simulink model "full_system"  (R2023b)
settings: Solver=VariableStepAuto  StartTime=0.0  StopTime=0.5  RelTol=1e-3
InitFcn:
  | init_full;
StopFcn:
  | PlotResults;
values from neighbouring files (symbols this model uses):
  Co = DCDC_Co*(10^-6)    [init_full.m]
  enc_offset = rand*2*pi    [init_full.m]
  id_KtMax = [0 -0.537821267309 -1.89621818766 -3.99825634278 -6.70443962951 -9.96764643107 -13.6215947621 -17.6528328359 -21.9311457912 -26.4320408854 -31.0887852115 -35.9145699207 ... (100 elements, 1x100)]    [Data_DCDC_converter.mat]
  IinMax = I_in_rated    [init_full.m]
  Imax = I_max    [init_full.m]
  iq_KtMax = [0 7.75916074359 15.4395487378 22.9882228687 30.3801205367 37.5897819046 44.6344030308 51.5031554736 58.229114561 64.8178001373 71.2942504703 77.6524098392 ... (100 elements, 1x100)]    [Data_DCDC_converter.mat]
  kid = 0.05*kpd*wb    [init_full.m]
  kii = 2106.71507358    [Data_DCDC_converter.mat]    (also in init_full.m = wzi*kpi)
  kiq = 0.05*kpq*wb    [init_full.m]
  kiv = 443.093490604    [Data_DCDC_converter.mat]    (also in init_full.m = kpv*wzv)
  kpd = wb*ld    [init_full.m]
  kpi = 1.75559589465    [Data_DCDC_converter.mat]    (also in init_full.m = wci*Lin)
  kpq = wb*lq    [init_full.m]
  kpv = 0.678584013175    [Data_DCDC_converter.mat]    (also in init_full.m = wcv*Co)
  lambda_m = F_m    [init_full.m]
  Lin = L    [init_full.m]
  p = 3    [Data_DCDC_converter.mat]
  Rs = 0.05    [Data_DCDC_converter.mat]
  Tau_d = 1.5*Ts    [init_full.m]
  TimeEnable = 5e-3    (= 0.005)    [init_full.m]
  Trise = 25e-3    (= 0.025)    [init_full.m]
  Ts = 1/fs    [init_full.m]
  Ts_inv = 1/fs_inv    [init_full.m]
  Vbat = DCDC_vbatt    [init_full.m]
  Vdc = Vdc_max    [init_full.m]
  VdcSetpoint = Vdc_max    [init_full.m]
  w_mech = 2459    [init_full.m]
undefined symbols (not defined in the file or in its folder): DiscIntNeverNeededParam, Ld_nom, Lq_nom, sigbuilder_block, T_KtMax
libraries: simulink x6, spsMeanLib x1
settings Model: Creator=giuse  LastModifiedBy=giuse

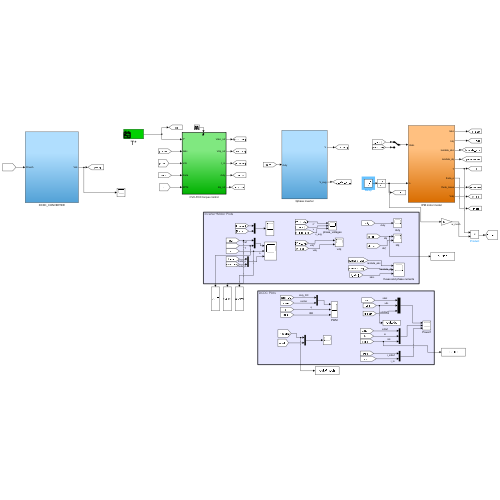
[thumbnail: Simulink's stored preview of the top-level diagram]
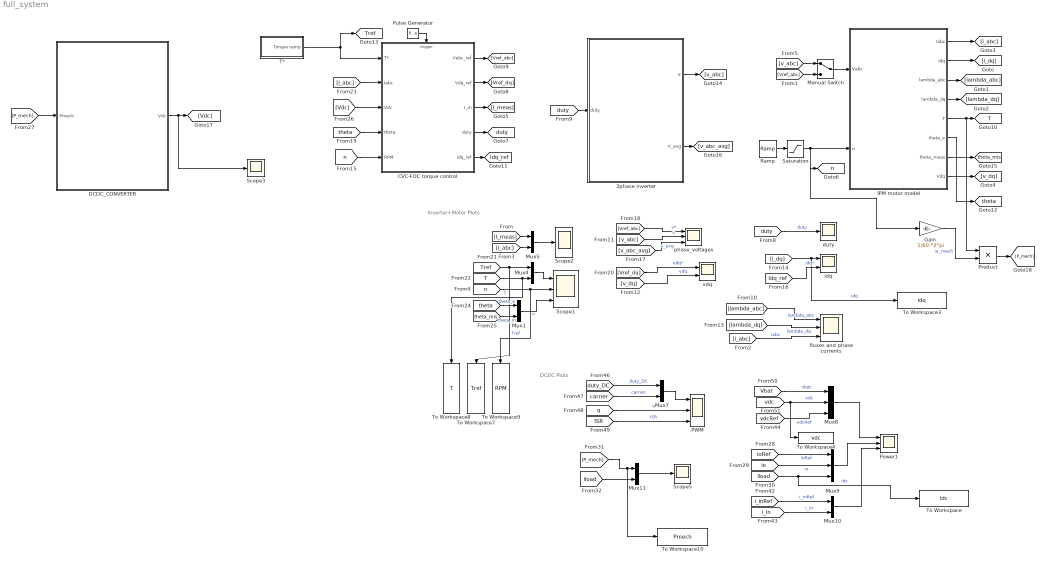
== system full_system ==
  note: DCDC Plots
  note: Inverter+Motor Plots
  3phase inverter : Subsystem
  CVC-FOC torque control : Subsystem
  DCDC_CONVERTER : Subsystem
  Gain : Gain  Gain=1/60 *2*pi
  IPM motor model : Subsystem
  Manual Switch : ManualSwitch
  Mux{1,4..5,7,10..11} (6 alike) : Mux  Inputs=2
  Mux8 : Mux  Inputs=3
  Mux9 : Mux  Inputs=3
  PWM : Scope  NumInputPorts=3
  Power1 : Scope  NumInputPorts=3
  Product : Product
  Pulse Generator : DiscretePulseGenerator  PulseType=Time based  Period=Ts_inv  PulseWidth=20
  Ramp : simulink/Sources/Ramp  slope=w_mech/0.3  start=0.1  InitialOutput=0
  Saturation : Saturate  UpperLimit=w_mech  LowerLimit=-100
  Scope1 : Scope  NumInputPorts=3
  Scope2 : Scope
  Scope3 : Scope
  Scope5 : Scope
  T* : Subsystem  Tag=STV Subsys  LoadFcn=sigbuilder_block('load');  StartFcn=sigbuilder_block('start');  StopFcn=sigbuilder_block('stop');  ClipboardFcn=sigbuilder_block('clipboard');  mask(Sigbuilder block){tuvar=[0:10]}
      mask help: Simulink:masks:SigbuilderBlock_MD
      mask init:
      | if ~strcmp(get_param(bdroot(gcbh),'SimulationStatus'),'stopped') tuvar = sigbuilder_block('maskInit'); end
      settings: CopyFcn=sigbuilder_block('copy');  DeleteFcn=sigbuilder_block('delete');  ModelCloseFcn=sigbuilder_block('modelClose');  PreSaveFcn=sigbuilder_block('preSave');  PauseFcn=sigbuilder_block('pause');  ContinueFcn=sigbuilder_block('continue');  NameChangeFcn=sigbuilder_block('namechange');  OpenFcn=sigbuilder_block('open',[5.4 30 1141.2 522.6 ]);  CloseFcn=sigbuilder_block('close');
      mask Display: plot(0, 0, 100, 100,[2, 2, 32, 32, 2], [68, 8, 8, 68, 68],[32, 2], [38, 38], [32, 19, 2],[53, 60, 44], [32, 17, 17, 2],[16, 16, 31, 31]);txt = getActiveGroup(gcbh);text(2, 100, txt,'verticalAlignment', 'top');
  To Workspace : ToWorkspace  VariableName=idc  SampleTime=-1
  To Workspace10 : ToWorkspace  VariableName=Pmech  SampleTime=-1
  To Workspace3 : ToWorkspace  VariableName=idq  SampleTime=-1
  To Workspace4 : ToWorkspace  VariableName=vdc  SampleTime=-1
  To Workspace7 : ToWorkspace  VariableName=Tref  SampleTime=-1
  To Workspace8 : ToWorkspace  VariableName=T  SampleTime=-1
  To Workspace9 : ToWorkspace  VariableName=RPM  SampleTime=-1
  duty : Scope
  fluxes and phase currents : Scope  NumInputPorts=3
  idq : Scope  NumInputPorts=2
  phase_voltages : Scope  NumInputPorts=3
  vdq : Scope  NumInputPorts=2
  tag scope: Idq_ref=global, T=global, Tref=global, duty=global, n=global, theta=global, theta_mis=global
  wires:
  [i_abc] -> CVC-FOC torque control/2(Iabc)
  [Vref_abc] -> phase_voltages/1  "v*"
  Pulse Generator/1 -> CVC-FOC torque control/Trigger
  CVC-FOC torque control/3(I_m) -> [I_meas]
  [v_abc] -> Manual Switch/1
  CVC-FOC torque control/5(Idq_ref) -> [Idq_ref]
  T*/1(Torque ramp) -> CVC-FOC torque control/1(T*), [Tref]
  IPM motor model/3(lambda_abc) -> [lambda_abc]
  CVC-FOC torque control/4(duty) -> [duty]
  [n] -> CVC-FOC torque control/5(RPM)
  [Idq_ref] -> idq/2  "idq*"
  [T] -> To Workspace8/1, Mux4/2  "T"
  [Vref_dq] -> vdq/1  "vdq*"
  [I_meas] -> Mux5/1
  3phase inverter/2(V_avg) -> [v_abc_avg]
  [i_dq] -> To Workspace3/1, idq/1  "idq"
  Manual Switch/1 -> IPM motor model/1(Vabc)
  [Vdc] -> CVC-FOC torque control/3(Vdc)
  Mux5/1 -> Scope2/1
  IPM motor model/1(Iabc) -> [i_abc]
  [i_abc] -> Mux5/2
  [Vref_abc] -> Manual Switch/2
  IPM motor model/8(Vdq) -> [v_dq]
  Mux4/1 -> Scope1/1
  CVC-FOC torque control/2(Vdq_ref) -> [Vref_dq]
  Saturation/1 -> [n], IPM motor model/2(n), Gain/1
  [v_abc] -> phase_voltages/2  "v"
  [Tref] -> Mux4/1, To Workspace7/1  "Tref"
  Ramp/1 -> Saturation/1
  [theta] -> CVC-FOC torque control/4(theta)
  IPM motor model/7(theta_meas) -> [theta_mis]
  IPM motor model/2(Idq) -> [i_dq]
  [theta_mis] -> Mux1/2  "theta_m"
  [duty] -> 3phase inverter/1(duty)
  CVC-FOC torque control/1(Vabc_ref) -> [Vref_abc]
  IPM motor model/6(theta_e) -> [theta]
  IPM motor model/5(T) -> Product/1, [T]
  [v_abc_avg] -> phase_voltages/3  "v_avg"
  [lambda_dq] -> fluxes and phase currents/2  "lambda_dq"
  [n] -> Scope1/2, To Workspace9/1  "n"
  [theta] -> Mux1/1  "theta_e"
  Mux1/1 -> Scope1/3
  IPM motor model/4(lambda_dq) -> [lambda_dq]
  3phase inverter/1(V) -> [v_abc]
  [v_dq] -> vdq/2  "vdq"
  [duty] -> duty/1  "duty"
  [lambda_abc] -> fluxes and phase currents/1  "lambda_abc"
  [i_abc] -> fluxes and phase currents/3  "iabc"
  Mux10/1 -> Power1/3
  [ioRef] -> Mux9/1  "ioRef"
  Mux7/1 -> PWM/1
  [i_inRef] -> Mux10/1  "i_inRef"
  [i_in] -> Mux10/2  "i_in"
  [carrier] -> Mux7/2  "carrier"
  [vdcRef] -> Mux8/3  "vdcRef"
  [ISR] -> PWM/3  "ISR"
  [Vbat] -> Mux8/1  "vbat"
  [q] -> PWM/2  "q"
  [iload] -> Mux9/3, To Workspace/1  "idc"
  [io] -> Mux9/2  "io"
  [vdc] -> To Workspace4/1, Mux8/2  "vdc"
  Mux8/1 -> Power1/1
  [duty_DC] -> Mux7/1  "duty_DC"
  Mux9/1 -> Power1/2
  DCDC_CONVERTER/1(Vdc) -> Scope3/1, [Vdc]
  Gain/1 -> Product/2  "w_mech"
  Product/1 -> [P_mech]
  [P_mech] -> DCDC_CONVERTER/1(Pmech)
  Mux11/1 -> Scope5/1
  [iload] -> Mux11/2
  [P_mech] -> To Workspace10/1, Mux11/1

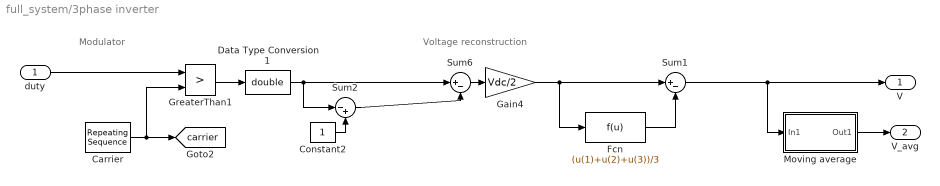
== system full_system/3phase inverter ==
  note: Modulator
  note: Voltage reconstruction
  duty : Inport
  Carrier : simulink/Sources/Repeating Sequence  rep_seq_t=[0 Ts/2 Ts]  rep_seq_y=[0 1 0]
  Constant2 : Constant
  Data Type Conversion1 : DataTypeConversion  OutDataTypeStr=double  SaturateOnIntegerOverflow=off  RndMeth=Floor
  Fcn : Fcn  Expr=(u(1)+u(2)+u(3))/3
  Gain4 : Gain  Gain=Vdc/2
  GreaterThan1 : RelationalOperator  Operator=>  OutDataTypeStr=boolean  RndMeth=Simplest  InputSameDT=off
  Moving average : Subsystem
  Sum1 : Sum  Inputs=|+-
  Sum2 : Sum  Inputs=|-+
  Sum6 : Sum  Inputs=|+-
  V : Outport  VectorParamsAs1DForOutWhenUnconnected=off
  V_avg : Outport  Port=2  VectorParamsAs1DForOutWhenUnconnected=off
  tag scope: carrier=global
  wires:
  GreaterThan1/1 -> Data Type Conversion1/1
  Moving average/1(Out1) -> V_avg/1
  Carrier/1 -> [carrier], GreaterThan1/2
  Data Type Conversion1/1 -> Sum2/1, Sum6/1
  Constant2/1 -> Sum2/2
  Sum6/1 -> Gain4/1
  duty/1 -> GreaterThan1/1
  Gain4/1 -> Fcn/1, Sum1/1
  Sum1/1 -> Moving average/1(In1), V/1
  Fcn/1 -> Sum1/2
  Sum2/1 -> Sum6/2

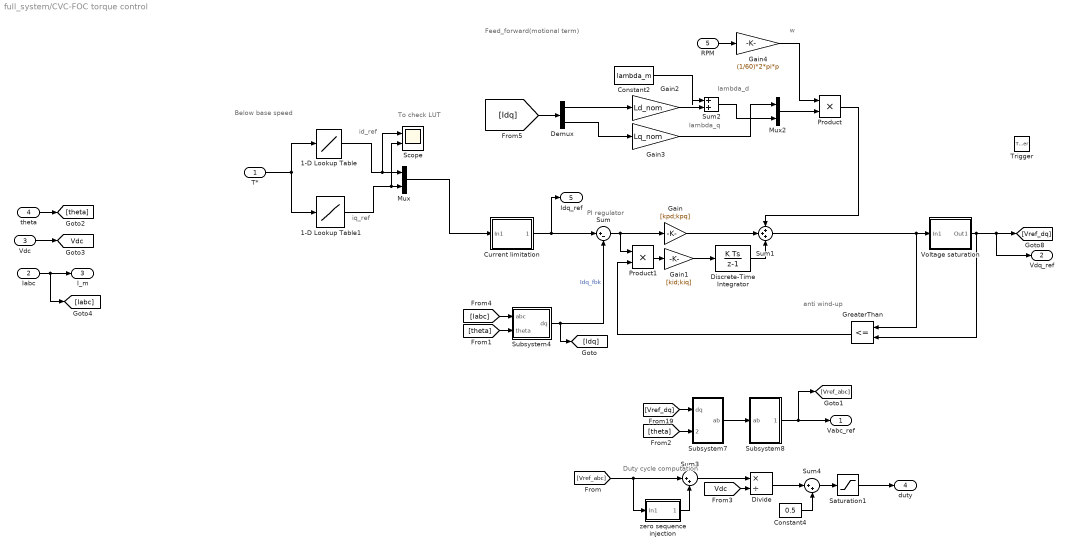
== system full_system/CVC-FOC torque control ==
  note: To check LUT
  note: Feed_forward(motional term)
  note: w
  note: lambda_q
  note: lambda_d
  note: iq_ref
  note: id_ref
  note: Below base speed
  note: anti wind-up
  note: PI regulator
  note: Duty cycle computation
  T* : Inport
  Iabc : Inport  Port=2
  Vdc : Inport  Port=3
  theta : Inport  Port=4
  RPM : Inport  Port=5
  Trigger : TriggerPort  VariantControl=Variant  PortDimensions=1
  1-D Lookup Table : Lookup_n-D  NumberOfTableDimensions=1  BreakpointsForDimension1=T_KtMax  Table=id_KtMax  InternalRulePriority=Speed  RndMeth=Simplest
  1-D Lookup Table1 : Lookup_n-D  NumberOfTableDimensions=1  BreakpointsForDimension1=T_KtMax  Table=iq_KtMax  InternalRulePriority=Speed  RndMeth=Simplest
  Constant2 : Constant  Value=lambda_m
  Constant4 : Constant  Value=0.5
  Current limitation : Subsystem
  Demux : Demux  Outputs=2
  Discrete-Time Integrator : DiscreteIntegrator  gainval=1  SampleTime=-1  ICPrevOutput=DiscIntNeverNeededParam  ICPrevScaledInput=DiscIntNeverNeededParam
  Divide : Product  Inputs=*/
  Gain : Gain  Gain=[kpd;kpq]
  Gain1 : Gain  Gain=[kid;kiq]
  Gain2 : Gain  Gain=Ld_nom
  Gain3 : Gain  Gain=Lq_nom
  Gain4 : Gain  Gain=(1/60)*2*pi*p
  GreaterThan : RelationalOperator  Operator=<=  OutDataTypeStr=boolean  RndMeth=Simplest  InputSameDT=off
  Mux : Mux  Inputs=2
  Mux2 : Mux  Inputs=2
  Product : Product
  Product1 : Product
  Saturation1 : Saturate  UpperLimit=1  LowerLimit=0
  Scope : Scope  NumInputPorts=2
  Subsystem4 : Subsystem
  Subsystem7 : Subsystem
  Subsystem8 : Subsystem
  Sum : Sum  Inputs=|+-
  Sum1 : Sum  Inputs=+++
  Sum2 : Sum  Inputs=|++
  Sum3 : Sum  Inputs=|++
  Sum4 : Sum  Inputs=|++
  Voltage saturation : Subsystem
  zero sequence injection : Subsystem
  Vabc_ref : Outport  VectorParamsAs1DForOutWhenUnconnected=off
  Vdq_ref : Outport  Port=2  VectorParamsAs1DForOutWhenUnconnected=off
  I_m : Outport  Port=3  VectorParamsAs1DForOutWhenUnconnected=off
  duty : Outport  Port=4  VectorParamsAs1DForOutWhenUnconnected=off
  Idq_ref : Outport  Port=5
  tag scope: Vdc=global
  wires:
  Subsystem7/1(ab) -> Subsystem8/1(ab)
  [Vref_dq] -> Subsystem7/1(dq)
  Subsystem8/1(abc) -> [Vref_abc], Vabc_ref/1
  Iabc/1 -> [Iabc], I_m/1
  Sum/1 -> Product1/1, Gain/1
  Gain1/1 -> Discrete-Time Integrator/1
  Saturation1/1 -> duty/1
  Constant4/1 -> Sum4/2
  zero sequence injection/1(Out1) -> Sum3/2
  Sum3/1 -> Divide/1
  [Vdc] -> Divide/2
  Sum4/1 -> Saturation1/1
  [Vref_abc] -> zero sequence injection/1(In1), Sum3/1
  Divide/1 -> Sum4/1
  theta/1 -> [theta]
  [theta] -> Subsystem7/2(theta)
  Subsystem4/1(dq) -> Sum/2, [Idq]  "Idq_fbk"
  Vdc/1 -> [Vdc]
  [theta] -> Subsystem4/2(theta)
  [Iabc] -> Subsystem4/1(abc)
  Sum1/1 -> Voltage saturation/1(In1), GreaterThan/1
  Product1/1 -> Gain1/1
  GreaterThan/1 -> Product1/2
  T*/1 -> 1-D Lookup Table1/1, 1-D Lookup Table/1
  1-D Lookup Table/1 -> Scope/1, Mux/1
  1-D Lookup Table1/1 -> Scope/2, Mux/2
  Current limitation/1(Idq_ref) -> Idq_ref/1, Sum/1
  Mux/1 -> Current limitation/1(In1)
  [Idq] -> Demux/1
  Demux/1 -> Gain2/1
  Gain2/1 -> Sum2/2
  Constant2/1 -> Sum2/1
  Demux/2 -> Gain3/1
  Sum2/1 -> Mux2/2
  Gain3/1 -> Mux2/1
  Mux2/1 -> Product/2
  RPM/1 -> Gain4/1
  Gain4/1 -> Product/1
  Discrete-Time Integrator/1 -> Sum1/3
  Gain/1 -> Sum1/2
  Product/1 -> Sum1/1
  Voltage saturation/1(Out1) -> [Vref_dq], Vdq_ref/1, GreaterThan/2

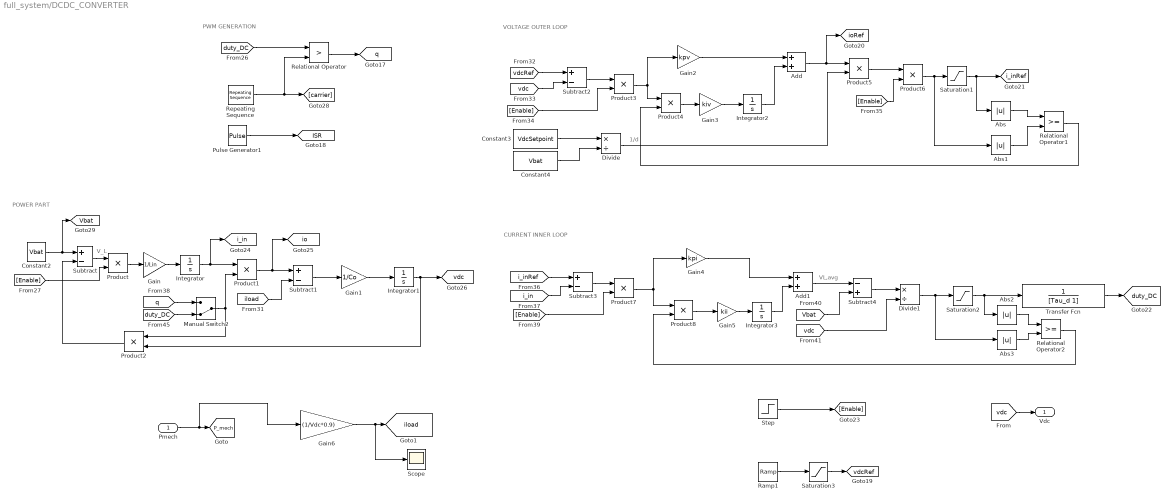
== system full_system/DCDC_CONVERTER ==
  note: V_L
  note: POWER PART
  note: PWM GENERATION
  note: CURRENT INNER LOOP
  note: VOLTAGE OUTER LOOP
  note: 1/d
  note: VL,avg
  Pmech : Inport
  Abs{,1..3} (4 alike) : Abs  SaturateOnIntegerOverflow=off
  Add : Sum
  Add1 : Sum
  Constant2 : Constant  Value=Vbat
  Constant3 : Constant  Value=VdcSetpoint
  Constant4 : Constant  Value=Vbat
  Divide : Product  Inputs=*/
  Divide1 : Product  Inputs=*/
  Gain : Gain  Gain=1/Lin
  Gain1 : Gain  Gain=1/Co
  Gain2 : Gain  Gain=kpv
  Gain3 : Gain  Gain=kiv
  Gain4 : Gain  Gain=kpi
  Gain5 : Gain  Gain=kii
  Gain6 : Gain  Gain=(1/Vdc*0.9)
  Integrator : Integrator
  Integrator1 : Integrator  InitialCondition=Vbat
  Integrator2 : Integrator
  Integrator3 : Integrator
  Manual Switch2 : ManualSwitch  CurrentSetting=0
  Product{,1..8} (9 alike) : Product
  Pulse Generator1 : DiscretePulseGenerator  PulseType=Time based  Period=Ts  PulseWidth=50
  Ramp1 : simulink/Sources/Ramp  slope=(VdcSetpoint-Vbat)/Trise  start=TimeEnable  InitialOutput=Vbat
  Relational Operator : RelationalOperator  Operator=>  RndMeth=Simplest  InputSameDT=off
  Relational Operator1 : RelationalOperator  RndMeth=Simplest
  Relational Operator2 : RelationalOperator  RndMeth=Simplest
  Repeating Sequence : simulink/Sources/Repeating Sequence  rep_seq_t=[0 Ts/2 Ts]  rep_seq_y=[0 1 0]
  Saturation1 : Saturate  UpperLimit=IinMax  LowerLimit=-IinMax
  Saturation2 : Saturate  UpperLimit=1  LowerLimit=0.1
  Saturation3 : Saturate  UpperLimit=VdcSetpoint  LowerLimit=Vbat
  Scope : Scope
  Step : Step  Time=TimeEnable  SampleTime=0
  Subtract{,1..3} (4 alike) : Sum  Inputs=+-
  Subtract4 : Sum  Inputs=-+
  Transfer Fcn : TransferFcn  Denominator=[Tau_d 1]
  Vdc : Outport
  tag scope: ISR=global, P_mech=global, Vbat=global, duty_DC=global, i_in=global, i_inRef=global, iload=global, io=global, ioRef=global, q=global, vdc=global, vdcRef=global
  wires:
  Transfer Fcn/1 -> [duty_DC]
  Manual Switch2/1 -> Product2/1, Product1/2
  Integrator1/1 -> [vdc], Product2/2
  Add1/1 -> Subtract4/1
  Subtract/1 -> Product/1
  Saturation3/1 -> [vdcRef]
  Saturation2/1 -> Transfer Fcn/1, Abs2/1
  Product6/1 -> Abs1/1, Saturation1/1
  Abs1/1 -> Relational Operator1/2
  [Enable] -> Product/2
  Subtract2/1 -> Product3/1
  Gain1/1 -> Integrator1/1
  Relational Operator2/1 -> Product8/2
  [Vbat] -> Subtract4/2
  Constant2/1 -> [Vbat], Subtract/1
  [i_inRef] -> Subtract3/1
  Subtract3/1 -> Product7/1
  Subtract1/1 -> Gain1/1
  Divide/1 -> Product5/2
  Product4/1 -> Gain3/1
  [i_in] -> Subtract3/2
  Ramp1/1 -> Saturation3/1
  Gain3/1 -> Integrator2/1
  Gain2/1 -> Add/1
  Constant3/1 -> Divide/1
  Integrator/1 -> Product1/1, [i_in]
  Subtract4/1 -> Divide1/1
  Pulse Generator1/1 -> [ISR]
  Product1/1 -> [io], Subtract1/1
  Product2/1 -> Subtract/2
  Gain/1 -> Integrator/1
  Product8/1 -> Gain5/1
  Product7/1 -> Product8/1, Gain4/1
  [duty_DC] -> Manual Switch2/2
  Divide1/1 -> Abs3/1, Saturation2/1
  [q] -> Manual Switch2/1
  [Enable] -> Product7/2
  [iload] -> Subtract1/2
  Relational Operator1/1 -> Product4/2
  [vdcRef] -> Subtract2/1
  Gain4/1 -> Add1/1
  [vdc] -> Divide1/2
  Repeating Sequence/1 -> [carrier], Relational Operator/2
  Abs3/1 -> Relational Operator2/2
  Product/1 -> Gain/1
  Relational Operator/1 -> [q]
  Abs/1 -> Relational Operator1/1
  [duty_DC] -> Relational Operator/1
  Abs2/1 -> Relational Operator2/1
  [Enable] -> Product6/2
  Gain5/1 -> Integrator3/1
  Step/1 -> [Enable]
  Integrator3/1 -> Add1/2
  Add/1 -> [ioRef], Product5/1
  Product5/1 -> Product6/1
  [vdc] -> Subtract2/2
  Saturation1/1 -> Abs/1, [i_inRef]
  Integrator2/1 -> Add/2
  Product3/1 -> Product4/1, Gain2/1
  [Enable] -> Product3/2
  Constant4/1 -> Divide/2
  [vdc] -> Vdc/1
  Pmech/1 -> Gain6/1, [P_mech]
  Gain6/1 -> Scope/1, [iload]

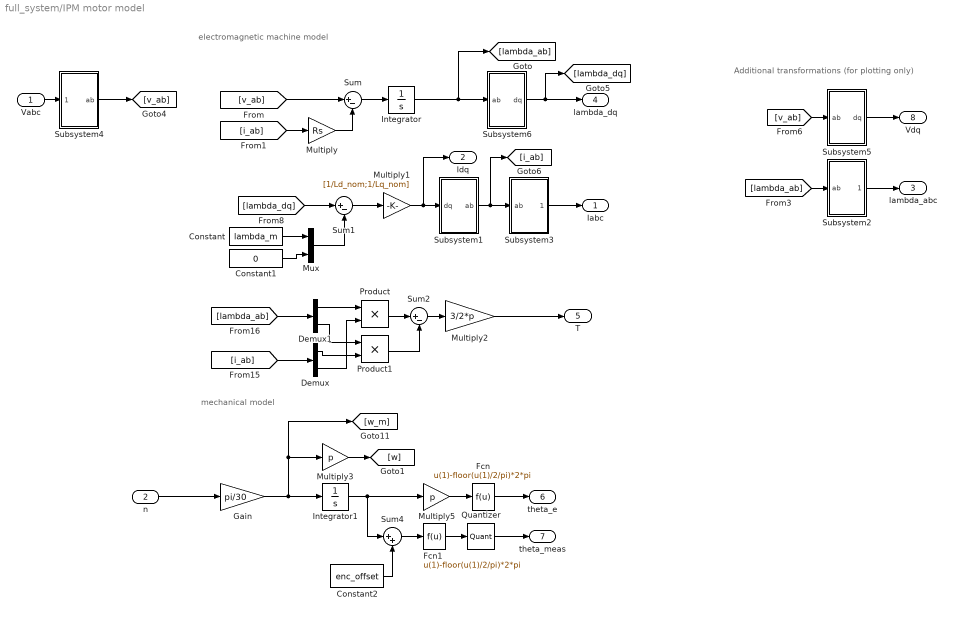
== system full_system/IPM motor model ==
  note: Additional transformations (for plotting only)
  note: mechanical model
  note: electromagnetic machine model
  Vabc : Inport
  n : Inport  Port=2
  Constant : Constant  Value=lambda_m
  Constant1 : Constant  Value=0
  Constant2 : Constant  Value=enc_offset
  Demux : Demux  Outputs=2
  Demux1 : Demux  Outputs=2
  Fcn : Fcn  Expr=u(1)-floor(u(1)/2/pi)*2*pi
  Fcn1 : Fcn  Expr=u(1)-floor(u(1)/2/pi)*2*pi
  Gain : Gain  Gain=pi/30
  Integrator : Integrator  InitialCondition=[lambda_m 0]
  Integrator1 : Integrator
  Multiply : Gain  Gain=Rs
  Multiply1 : Gain  Gain=[1/Ld_nom;1/Lq_nom]
  Multiply2 : Gain  Gain=3/2*p
  Multiply3 : Gain  Gain=p
  Multiply5 : Gain  Gain=p
  Mux : Mux  Inputs=2
  Product : Product
  Product1 : Product
  Quantizer : Quantizer  QuantizationInterval=2*pi/2048
  Subsystem1 : Subsystem
  Subsystem2 : Subsystem
  Subsystem3 : Subsystem
  Subsystem4 : Subsystem
  Subsystem5 : Subsystem
  Subsystem6 : Subsystem
  Sum : Sum  Inputs=|+-
  Sum1 : Sum  Inputs=|+-
  Sum2 : Sum  Inputs=|+-
  Sum4 : Sum  Inputs=|++
  Iabc : Outport  VectorParamsAs1DForOutWhenUnconnected=off
  Idq : Outport  Port=2  VectorParamsAs1DForOutWhenUnconnected=off
  lambda_abc : Outport  Port=3  VectorParamsAs1DForOutWhenUnconnected=off
  lambda_dq : Outport  Port=4  VectorParamsAs1DForOutWhenUnconnected=off
  T : Outport  Port=5  VectorParamsAs1DForOutWhenUnconnected=off
  theta_e : Outport  Port=6  VectorParamsAs1DForOutWhenUnconnected=off
  theta_meas : Outport  Port=7  VectorParamsAs1DForOutWhenUnconnected=off
  Vdq : Outport  Port=8  VectorParamsAs1DForOutWhenUnconnected=off
  wires:
  Integrator1/1 -> Multiply5/1, Sum4/1
  [v_ab] -> Sum/1
  [i_ab] -> Demux/1
  Fcn1/1 -> Quantizer/1
  [lambda_ab] -> Demux1/1
  Multiply/1 -> Sum/2
  Quantizer/1 -> theta_meas/1
  Integrator/1 -> Subsystem6/1(ab), [lambda_ab]
  Sum/1 -> Integrator/1
  Product/1 -> Sum2/1
  Subsystem4/1(ab) -> [v_ab]
  Subsystem6/1(dq) -> [lambda_dq], lambda_dq/1
  [lambda_dq] -> Sum1/1
  Subsystem5/1(dq) -> Vdq/1
  Sum1/1 -> Multiply1/1
  [v_ab] -> Subsystem5/1(ab)
  Fcn/1 -> theta_e/1
  Product1/1 -> Sum2/2
  Vabc/1 -> Subsystem4/1(abc)
  Multiply5/1 -> Fcn/1
  Subsystem1/1(ab) -> Subsystem3/1(ab), [i_ab]
  Multiply1/1 -> Idq/1, Subsystem1/1(dq)
  Sum4/1 -> Fcn1/1
  Gain/1 -> Integrator1/1, Multiply3/1, [w_m]
  Demux1/1 -> Product/1
  Demux/2 -> Product/2
  Demux1/2 -> Product1/1
  [lambda_ab] -> Subsystem2/1(ab)
  Demux/1 -> Product1/2
  [i_ab] -> Multiply/1
  Constant/1 -> Mux/1
  Constant1/1 -> Mux/2
  Mux/1 -> Sum1/2
  Sum2/1 -> Multiply2/1
  Constant2/1 -> Sum4/2
  Multiply2/1 -> T/1
  Subsystem3/1(abc) -> Iabc/1
  Subsystem2/1(abc) -> lambda_abc/1
  n/1 -> Gain/1
  Multiply3/1 -> [w]

== system full_system/T* ==
  Demux : Demux  Tag=STV Demux  Outputs=1
      settings: DisplayOption=none
  FromWs : FromWorkspace  Tag=STV FromWs  VariableName=tuvar
      SigBuilderData=|
      | common.afterFinalStr = 'Extrapolate'
      | common.sampleTime = 0
      | dataSet.timeRange = [0 3]
      | dataSet.name = 'T*'
      | sbobj.Groups.Name = 'T*'
      | sbobj.Groups.Signals.Name = 'Torque ramp'
      | sbobj.Groups.Signals.XData = [0 0.3 0.3 3]
      | sbobj.Groups.Signals.YData = [0 100 100 100]
      | sbobj.Groups.TimeRange = [0 3]
  Torque ramp : Outport  Tag=STV Outport
  wires:
  FromWs/1 -> Demux/1
  Demux/1 -> Torque ramp/1

== system full_system/3phase inverter/Moving average ==
  In1 : Inport
  Mean1 : spsMeanLib/Mean  Freq=fs  Vinit=0  Ts=0
  Out1 : Outport  VectorParamsAs1DForOutWhenUnconnected=off
  wires:
  In1/1 -> Mean1/1
  Mean1/1 -> Out1/1

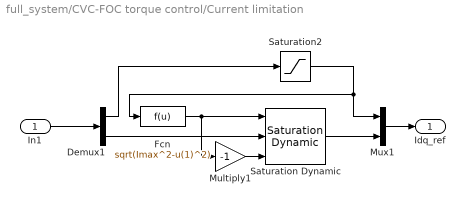
== system full_system/CVC-FOC torque control/Current limitation ==
  In1 : Inport
  Demux1 : Demux  Outputs=2
  Fcn : Fcn  Expr=sqrt(Imax^2-u(1)^2)
  Multiply1 : Gain  Gain=-1
  Mux1 : Mux  Inputs=2
  Saturation Dynamic : simulink/Discontinuities/Saturation Dynamic  OutMin=[]  OutMax=[]  OutDataTypeStr=Inherit: Same as second input  OutDataType=fixdt(1, 16)  OutScaling=2^-10  DoSatur=off
  Saturation2 : Saturate  UpperLimit=Imax  LowerLimit=-Imax
  Idq_ref : Outport  VectorParamsAs1DForOutWhenUnconnected=off
  wires:
  In1/1 -> Demux1/1
  Demux1/2 -> Saturation Dynamic/2
  Saturation2/1 -> Mux1/1, Fcn/1
  Mux1/1 -> Idq_ref/1
  Multiply1/1 -> Saturation Dynamic/3
  Demux1/1 -> Saturation2/1
  Fcn/1 -> Saturation Dynamic/1, Multiply1/1
  Saturation Dynamic/1 -> Mux1/2

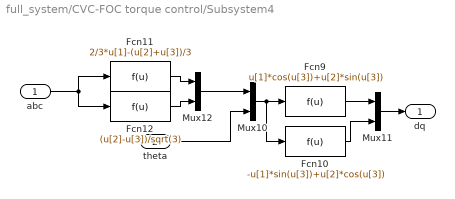
== system full_system/CVC-FOC torque control/Subsystem4 ==
  abc : Inport
  theta : Inport  Port=2
  Fcn10 : Fcn  Expr=-u[1]*sin(u[3])+u[2]*cos(u[3])
  Fcn11 : Fcn  Expr=2/3*u[1]-(u[2]+u[3])/3
  Fcn12 : Fcn  Expr=(u[2]-u[3])/sqrt(3)
  Fcn9 : Fcn  Expr=u[1]*cos(u[3])+u[2]*sin(u[3])
  Mux10 : Mux  Inputs=2
  Mux11 : Mux  Inputs=2
  Mux12 : Mux  Inputs=2
  dq : Outport  VectorParamsAs1DForOutWhenUnconnected=off
  wires:
  Fcn12/1 -> Mux12/2
  abc/1 -> Fcn12/1, Fcn11/1
  Fcn11/1 -> Mux12/1
  Fcn9/1 -> Mux11/1
  Mux10/1 -> Fcn10/1, Fcn9/1
  Mux12/1 -> Mux10/1
  Mux11/1 -> dq/1
  Fcn10/1 -> Mux11/2
  theta/1 -> Mux10/2

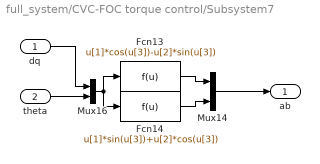
== system full_system/CVC-FOC torque control/Subsystem7 ==
  dq : Inport
  theta : Inport  Port=2
  Fcn13 : Fcn  Expr=u[1]*cos(u[3])-u[2]*sin(u[3])
  Fcn14 : Fcn  Expr=u[1]*sin(u[3])+u[2]*cos(u[3])
  Mux14 : Mux  Inputs=2
  Mux16 : Mux  Inputs=2
  ab : Outport  VectorParamsAs1DForOutWhenUnconnected=off
  wires:
  Fcn13/1 -> Mux14/1
  Mux16/1 -> Fcn13/1, Fcn14/1
  Fcn14/1 -> Mux14/2
  dq/1 -> Mux16/1
  Mux14/1 -> ab/1
  theta/1 -> Mux16/2

== system full_system/CVC-FOC torque control/Subsystem8 ==
  ab : Inport
  Fcn15 : Fcn  Expr=u[1]
  Fcn16 : Fcn  Expr=-u[1]*0.5+u[2]*sqrt(3)/2
  Fcn17 : Fcn  Expr=-u[1]*0.5-u[2]*sqrt(3)/2
  Mux15 : Mux  Inputs=3
  abc : Outport  VectorParamsAs1DForOutWhenUnconnected=off
  wires:
  Mux15/1 -> abc/1
  Fcn17/1 -> Mux15/3
  Fcn15/1 -> Mux15/1
  Fcn16/1 -> Mux15/2
  ab/1 -> Fcn16/1, Fcn17/1, Fcn15/1

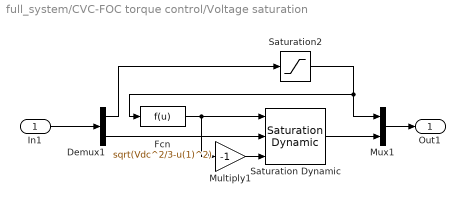
== system full_system/CVC-FOC torque control/Voltage saturation ==
  In1 : Inport
  Demux1 : Demux  Outputs=2
  Fcn : Fcn  Expr=sqrt(Vdc^2/3-u(1)^2)
  Multiply1 : Gain  Gain=-1
  Mux1 : Mux  Inputs=2
  Saturation Dynamic : simulink/Discontinuities/Saturation Dynamic  OutMin=[]  OutMax=[]  OutDataTypeStr=Inherit: Same as second input  OutDataType=fixdt(1, 16)  OutScaling=2^-10  DoSatur=off
  Saturation2 : Saturate  UpperLimit=Vdc/sqrt(3)  LowerLimit=-Vdc/sqrt(3)
  Out1 : Outport  VectorParamsAs1DForOutWhenUnconnected=off
  wires:
  Saturation Dynamic/1 -> Mux1/2
  Fcn/1 -> Multiply1/1, Saturation Dynamic/1
  Demux1/1 -> Saturation2/1
  Multiply1/1 -> Saturation Dynamic/3
  Mux1/1 -> Out1/1
  Saturation2/1 -> Fcn/1, Mux1/1
  Demux1/2 -> Saturation Dynamic/2
  In1/1 -> Demux1/1

== system full_system/CVC-FOC torque control/zero sequence injection ==
  In1 : Inport
  Fcn : Fcn  Expr=-0.5*(u(1)+u(2))
  Max : MinMax  Function=max
  Max1 : MinMax
  Mux7 : Mux  Inputs=2
  Out1 : Outport  VectorParamsAs1DForOutWhenUnconnected=off
  wires:
  Mux7/1 -> Fcn/1
  In1/1 -> Max1/1, Max/1
  Max1/1 -> Mux7/2
  Max/1 -> Mux7/1
  Fcn/1 -> Out1/1

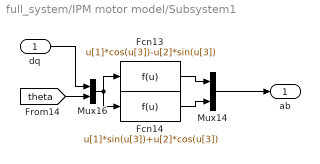
== system full_system/IPM motor model/Subsystem1 ==
  dq : Inport
  Fcn13 : Fcn  Expr=u[1]*cos(u[3])-u[2]*sin(u[3])
  Fcn14 : Fcn  Expr=u[1]*sin(u[3])+u[2]*cos(u[3])
  Mux14 : Mux  Inputs=2
  Mux16 : Mux  Inputs=2
  ab : Outport  VectorParamsAs1DForOutWhenUnconnected=off
  wires:
  Mux14/1 -> ab/1
  dq/1 -> Mux16/1
  Fcn14/1 -> Mux14/2
  Mux16/1 -> Fcn14/1, Fcn13/1
  Fcn13/1 -> Mux14/1
  [theta] -> Mux16/2

== system full_system/IPM motor model/Subsystem2 ==
  ab : Inport
  Fcn15 : Fcn  Expr=u[1]
  Fcn16 : Fcn  Expr=-u[1]*0.5+u[2]*sqrt(3)/2
  Fcn17 : Fcn  Expr=-u[1]*0.5-u[2]*sqrt(3)/2
  Mux15 : Mux  Inputs=3
  abc : Outport  VectorParamsAs1DForOutWhenUnconnected=off
  wires:
  Mux15/1 -> abc/1
  Fcn17/1 -> Mux15/3
  Fcn15/1 -> Mux15/1
  Fcn16/1 -> Mux15/2
  ab/1 -> Fcn16/1, Fcn17/1, Fcn15/1

== system full_system/IPM motor model/Subsystem3 ==
  ab : Inport
  Fcn15 : Fcn  Expr=u[1]
  Fcn16 : Fcn  Expr=-u[1]*0.5+u[2]*sqrt(3)/2
  Fcn17 : Fcn  Expr=-u[1]*0.5-u[2]*sqrt(3)/2
  Mux15 : Mux  Inputs=3
  abc : Outport  VectorParamsAs1DForOutWhenUnconnected=off
  wires:
  ab/1 -> Fcn15/1, Fcn17/1, Fcn16/1
  Fcn16/1 -> Mux15/2
  Fcn15/1 -> Mux15/1
  Fcn17/1 -> Mux15/3
  Mux15/1 -> abc/1

== system full_system/IPM motor model/Subsystem4 ==
  abc : Inport
  Fcn11 : Fcn  Expr=2/3*u[1]-(u[2]+u[3])/3
  Fcn12 : Fcn  Expr=(u[2]-u[3])/sqrt(3)
  Mux12 : Mux  Inputs=2
  ab : Outport  VectorParamsAs1DForOutWhenUnconnected=off
  wires:
  Mux12/1 -> ab/1
  Fcn12/1 -> Mux12/2
  abc/1 -> Fcn12/1, Fcn11/1
  Fcn11/1 -> Mux12/1

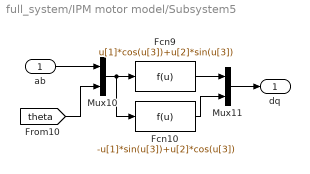
== system full_system/IPM motor model/Subsystem5 ==
  ab : Inport
  Fcn10 : Fcn  Expr=-u[1]*sin(u[3])+u[2]*cos(u[3])
  Fcn9 : Fcn  Expr=u[1]*cos(u[3])+u[2]*sin(u[3])
  Mux10 : Mux  Inputs=2
  Mux11 : Mux  Inputs=2
  dq : Outport  VectorParamsAs1DForOutWhenUnconnected=off
  wires:
  ab/1 -> Mux10/1
  [theta] -> Mux10/2
  Fcn9/1 -> Mux11/1
  Mux10/1 -> Fcn10/1, Fcn9/1
  Fcn10/1 -> Mux11/2
  Mux11/1 -> dq/1

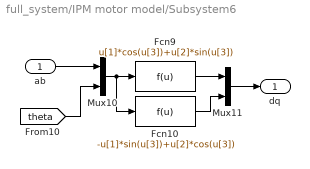
== system full_system/IPM motor model/Subsystem6 ==
  ab : Inport
  Fcn10 : Fcn  Expr=-u[1]*sin(u[3])+u[2]*cos(u[3])
  Fcn9 : Fcn  Expr=u[1]*cos(u[3])+u[2]*sin(u[3])
  Mux10 : Mux  Inputs=2
  Mux11 : Mux  Inputs=2
  dq : Outport  VectorParamsAs1DForOutWhenUnconnected=off
  wires:
  Mux11/1 -> dq/1
  Fcn10/1 -> Mux11/2
  Mux10/1 -> Fcn9/1, Fcn10/1
  Fcn9/1 -> Mux11/1
  [theta] -> Mux10/2
  ab/1 -> Mux10/1
